simulink model "autopilot_full"  (R2016b)
settings: Solver=VariableStepAuto  StartTime=0.0  StopTime=sim_time  RelTol=1e-3
values from neighbouring files (symbols this model uses):
  A = [ -0.322 0.052 0.028 -1.12 0.002 ... (first row only)    [autopilot_constants.m]
  B = [ 0 0 0 0 10]'    [autopilot_constants.m]
  C = [0 0 0 1 0 ... (first row only)    [autopilot_constants.m]
  d = 33*deg2rad    [run_task_2f.m]
  D = [0 0 0 0]'    [autopilot_constants.m]
  delta_a_max = 25*deg2rad    (= 0.436332312999)    [autopilot_constants.m]
  g = 9.81    [autopilot_constants.m]
  integratorlowerbound = -inf    [run_task_2f.m]
  integratorupperbound = inf    [run_task_2f.m]
  k_d_phi = (2*zeta_phi*omega_n_phi - a_phi_1) / a_phi_2    [autopilot_constants.m]
  k_i_chi = omega_n_chi^2*V_g/g    [autopilot_constants.m]    (also in prob2b.m = omega_n_chi^2 * V_g / g)
  k_i_phi = -.1    (= -0.1)    [autopilot_constants.m]
  k_p_chi = 2*zeta_chi*omega_n_chi*V_g/g    [autopilot_constants.m]    (also in prob2b.m = 2 * zeta_chi * omega_n_chi * V_g / g)
  k_p_phi = delta_a_max / e_phi_max * sign(a_phi_2)    [autopilot_constants.m]
  V_g = 637/3.6    (= 176.944444444)    [autopilot_constants.m]
libraries: aerolibconvert2 x1
settings Model: Creator=Alexandra  LastModifiedBy=HenningWard

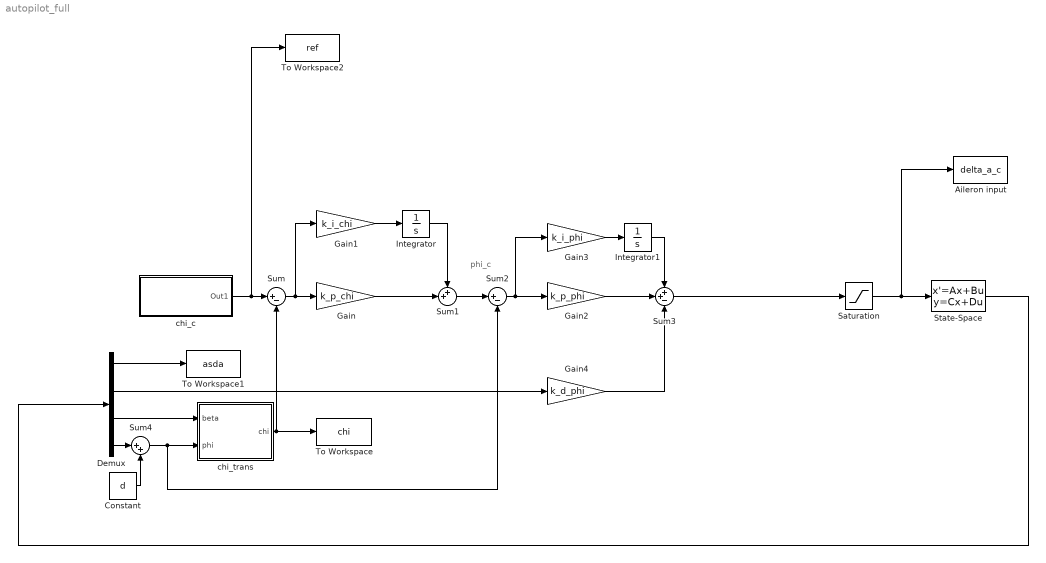
== system autopilot_full ==
  note: phi_c
  Aileron input : ToWorkspace  VariableName=delta_a_c  SaveFormat=Structure With Time  SampleTime=-1
  Constant : Constant  Value=d
  Demux : Demux
  Gain : Gain  Gain=k_p_chi
  Gain1 : Gain  Gain=k_i_chi
  Gain2 : Gain  Gain=k_p_phi
  Gain3 : Gain  Gain=k_i_phi
  Gain4 : Gain  Gain=k_d_phi
  Integrator : Integrator  UpperSaturationLimit=integratorupperbound  LowerSaturationLimit=integratorlowerbound
  Integrator1 : Integrator  LimitOutput=on  UpperSaturationLimit=integratorupperbound  LowerSaturationLimit=integratorlowerbound
  Saturation : Saturate  UpperLimit=delta_a_max  LowerLimit=-delta_a_max
  State-Space : StateSpace  A=A  B=B  C=C  D=D  X0=0
  Sum : Sum  Inputs=|+-
  Sum1 : Sum  Inputs=++|
  Sum2 : Sum  Inputs=|+-
  Sum3 : Sum  Inputs=++-
  Sum4 : Sum  Inputs=|++
  To Workspace : ToWorkspace  VariableName=chi  SaveFormat=Structure With Time  SampleTime=-1
  To Workspace1 : ToWorkspace  VariableName=asda  SaveFormat=Structure With Time  SampleTime=-1
  To Workspace2 : ToWorkspace  VariableName=ref  SaveFormat=Structure With Time  SampleTime=-1
  chi_c : Subsystem
  chi_trans : Subsystem
  wires:
  chi_c/1(Out1) -> To Workspace2/1, Sum/1
  Sum/1 -> Gain1/1, Gain/1
  Gain1/1 -> Integrator/1
  Gain/1 -> Sum1/2
  Integrator/1 -> Sum1/1
  Sum1/1 -> Sum2/1
  Sum2/1 -> Gain3/1, Gain2/1
  Gain3/1 -> Integrator1/1
  Integrator1/1 -> Sum3/1
  Gain2/1 -> Sum3/2
  Gain4/1 -> Sum3/3
  Sum3/1 -> Saturation/1
  Saturation/1 -> State-Space/1, Aileron input/1
  State-Space/1 -> Demux/1
  Demux/2 -> Gain4/1
  Demux/3 -> chi_trans/1(beta)
  chi_trans/1(chi) -> To Workspace/1, Sum/2
  Demux/1 -> To Workspace1/1
  Demux/4 -> Sum4/1
  Sum4/1 -> Sum2/2, chi_trans/2(phi)
  Constant/1 -> Sum4/2

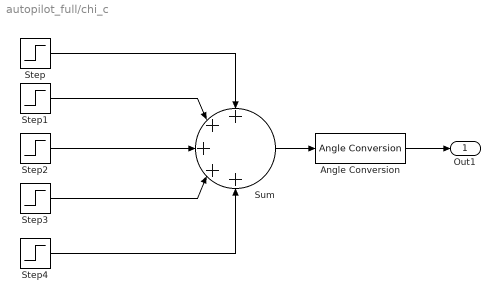
== system autopilot_full/chi_c ==
  Angle Conversion : aerolibconvert2/Angle Conversion  IU=deg  OU=rad
  Step : Step  Time=0  After=0  SampleTime=0
  Step1 : Step  Time=100  After=2  SampleTime=0
  Step2 : Step  Time=200  After=4  SampleTime=0
  Step3 : Step  Time=300  After=6  SampleTime=0
  Step4 : Step  Time=400  After=8  SampleTime=0
  Sum : Sum  Inputs=+++++
  Out1 : Outport
  wires:
  Step2/1 -> Sum/3
  Step1/1 -> Sum/2
  Step/1 -> Sum/1
  Step3/1 -> Sum/4
  Step4/1 -> Sum/5
  Sum/1 -> Angle Conversion/1
  Angle Conversion/1 -> Out1/1

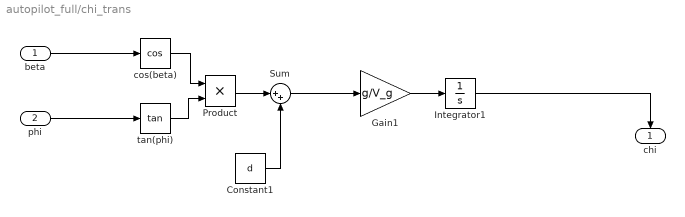
== system autopilot_full/chi_trans ==
  beta : Inport
  phi : Inport  Port=2
  Constant1 : Constant  Value=d
  Gain1 : Gain  Gain=g/V_g
  Integrator1 : Integrator
  Product : Product
  Sum : Sum  Inputs=|++
  cos(beta) : Trigonometry  Operator=cos
  tan(phi) : Trigonometry  Operator=tan
  chi : Outport
  wires:
  phi/1 -> tan(phi)/1
  Integrator1/1 -> chi/1
  beta/1 -> cos(beta)/1
  tan(phi)/1 -> Product/2
  cos(beta)/1 -> Product/1
  Gain1/1 -> Integrator1/1
  Product/1 -> Sum/1
  Sum/1 -> Gain1/1
  Constant1/1 -> Sum/2
